simulink model "pcssp_PowerSupplies"  (R2020b)
settings: Solver=VariableStepAuto  StartTime=0.0  StopTime=10.0  RelTol=1e-3
model workspace (MAT data in the model file):
  PS_tp = Simulink.Parameter
  PS_tp.Value.currentLim = [0 55000 200000]
  PS_tp.Value.voltageLim = [1200 1050 1050]
  PS_tp.Value.VS3Vup = 2300
  PS_tp.Value.VS3Vlow = -2300
  PS_tp.DataType = 'struct'
  PS_tp.Dimensions = [1 1]
undefined symbols (not defined in the file or in its folder): PS_fp
settings Model: DataDictionary=pcssp_PowerSupplies.sldd  ParameterArgumentNames=PS_tp  OrderedModelArguments=off  Creator=ravenst1  LastModifiedBy=ravenst1
settings DebuggingCC: MergeDetectMultiDrivingBlocksExec=none
settings ModelReferenceCC: PropagateSignalLabelsOutOfModel=off

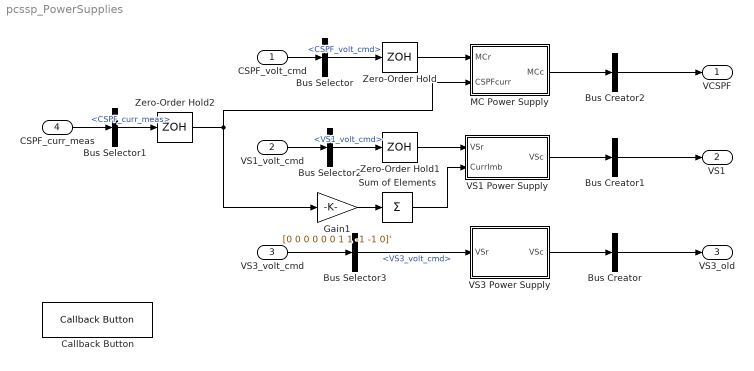
== system pcssp_PowerSupplies ==
  CSPF_volt_cmd : Inport  OutDataTypeStr=Bus: pcssp_PS_CSPF_volt_cmd  SampleTime=PS_fp.timing.dt
  VS1_volt_cmd : Inport  Port=2  OutDataTypeStr=Bus: pcssp_PS_VS1_volt_cmd  SampleTime=PS_fp.timing.dt
  VS3_volt_cmd : Inport  Port=3  OutDataTypeStr=Bus: pcssp_PS_VS3_volt_cmd  SampleTime=PS_fp.timing.dt
  CSPF_curr_meas : Inport  Port=4  OutDataTypeStr=Bus: pcssp_PS_CSPF_curr_meas  SampleTime=PS_fp.timing.dt
  Bus Creator : BusCreator  Inputs=1  OutDataTypeStr=Bus: pcssp_PS_VS3
      settings: InheritFromInputs=off
  Bus Creator1 : BusCreator  Inputs=1  OutDataTypeStr=Bus: pcssp_PS_VS1
      settings: InheritFromInputs=off
  Bus Creator2 : BusCreator  Inputs=1  OutDataTypeStr=Bus: pcssp_PS_VCSPF
      settings: InheritFromInputs=off
  Bus Selector : BusSelector  OutputSignals=CSPF_volt_cmd
  Bus Selector1 : BusSelector  OutputSignals=CSPF_curr_meas
  Bus Selector2 : BusSelector  OutputSignals=VS1_volt_cmd
  Bus Selector3 : BusSelector  OutputSignals=VS3_volt_cmd
  Callback Button : CallbackButton  ButtonText=Click for Module Documentation
      settings: ClickFcn=web(['file:///' which('PowerSupplies.html')])
  Gain1 : Gain  Gain=[0 0 0 0 0 0 1 1 -1 -1 0]'
  MC Power Supply : Subsystem
  Sum of Elements : Sum  Inputs=+
  VS1 Power Supply : Subsystem
  VS3 Power Supply : Subsystem
  Zero-Order Hold : ZeroOrderHold  SampleTime=PS_fp.timing.dt
  Zero-Order Hold1 : ZeroOrderHold  SampleTime=PS_fp.timing.dt
  Zero-Order Hold2 : ZeroOrderHold  SampleTime=PS_fp.timing.dt
  VCSPF : Outport  OutDataTypeStr=Bus: pcssp_PS_VCSPF
  VS1 : Outport  Port=2  OutDataTypeStr=Bus: pcssp_PS_VS1
  VS3_old : Outport  Port=3  OutDataTypeStr=Bus: pcssp_PS_VS3
  wires:
  VS3_volt_cmd/1 -> Bus Selector3/1
  Zero-Order Hold1/1 -> VS1 Power Supply/1(VSr)
  Sum of Elements/1 -> VS1 Power Supply/2(CurrImb)
  CSPF_curr_meas/1 -> Bus Selector1/1
  Zero-Order Hold2/1 -> Gain1/1, MC Power Supply/2(CSPFcurr)
  Zero-Order Hold/1 -> MC Power Supply/1(MCr)
  Gain1/1 -> Sum of Elements/1
  Bus Creator/1 -> VS3_old/1
  VS3 Power Supply/1(VSc) -> Bus Creator/1
  VS1 Power Supply/1(VSc) -> Bus Creator1/1
  Bus Creator1/1 -> VS1/1
  MC Power Supply/1(MCc) -> Bus Creator2/1
  Bus Creator2/1 -> VCSPF/1
  CSPF_volt_cmd/1 -> Bus Selector/1
  Bus Selector/1 -> Zero-Order Hold/1  "<CSPF_volt_cmd>"
  Bus Selector1/1 -> Zero-Order Hold2/1  "<CSPF_curr_meas>"
  VS1_volt_cmd/1 -> Bus Selector2/1
  Bus Selector2/1 -> Zero-Order Hold1/1  "<VS1_volt_cmd>"
  Bus Selector3/1 -> VS3 Power Supply/1(VSr)  "<VS3_volt_cmd>"

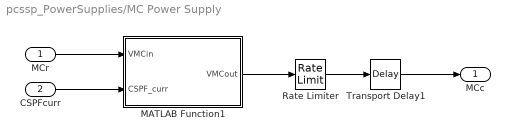
== system pcssp_PowerSupplies/MC Power Supply ==
  MCr : Inport
  CSPFcurr : Inport  Port=2
  MATLAB Function1 : MATLAB Function  TreatAsAtomicUnit=on  mask{currentLim=PS_tp.currentLim, voltageLim=PS_tp.voltageLim, nMConverters=PS_fp.nMConverters}
      mask prompts: currentLim "Current limits"; voltageLim "Voltage limits"; nMConverters "Number of CS/PF converters"
  Rate Limiter : RateLimiter  RisingSlewLimit=PS_fp.VMCpositiveSR  FallingSlewLimit=PS_fp.VMCnegativeSR  SampleTimeMode=inherited
  Transport Delay1 : TransportDelay  DelayTime=PS_fp.VMCtaud
  MCc : Outport
  wires:
  MCr/1 -> MATLAB Function1/1(VMCin)
  CSPFcurr/1 -> MATLAB Function1/2(CSPF_curr)
  MATLAB Function1/1(VMCout) -> Rate Limiter/1
  Rate Limiter/1 -> Transport Delay1/1
  Transport Delay1/1 -> MCc/1

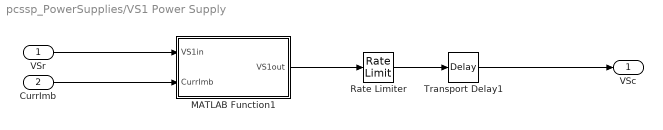
== system pcssp_PowerSupplies/VS1 Power Supply ==
  VSr : Inport
  CurrImb : Inport  Port=2
  MATLAB Function1 : MATLAB Function  TreatAsAtomicUnit=on  mask{currentLim=PS_tp.currentLim, voltageLim=PS_tp.voltageLim, nVS1Converters=PS_fp.nVS1Converters}
      mask prompts: currentLim "Current limit"; voltageLim "Voltage limit"; nVS1Converters "Number of VS1 converters"
  Rate Limiter : RateLimiter  RisingSlewLimit=PS_fp.VS1positiveSR  FallingSlewLimit=PS_fp.VS1negativeSR  SampleTimeMode=inherited
  Transport Delay1 : TransportDelay  DelayTime=PS_fp.VS1taud
  VSc : Outport
  wires:
  CurrImb/1 -> MATLAB Function1/2(CurrImb)
  VSr/1 -> MATLAB Function1/1(VS1in)
  Transport Delay1/1 -> VSc/1
  MATLAB Function1/1(VS1out) -> Rate Limiter/1
  Rate Limiter/1 -> Transport Delay1/1

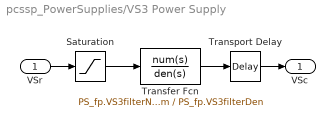
== system pcssp_PowerSupplies/VS3 Power Supply ==
  VSr : Inport
  Saturation : Saturate  UpperLimit=PS_tp.VS3Vup  LowerLimit=PS_tp.VS3Vlow
  Transfer Fcn : TransferFcn  Numerator=PS_fp.VS3filterNum  Denominator=PS_fp.VS3filterDen
  Transport Delay : TransportDelay  DelayTime=PS_fp.VS3taud
  VSc : Outport
  wires:
  VSr/1 -> Saturation/1
  Transport Delay/1 -> VSc/1
  Transfer Fcn/1 -> Transport Delay/1
  Saturation/1 -> Transfer Fcn/1

== matlab function pcssp_PowerSupplies/VS1 Power Supply/MATLAB Function1 ==
  data: VS1in input; VS1out output; CurrImb input; currentLim parameter; voltageLim parameter; nVS1Converters parameter
function VS1out  = fcn(VS1in, CurrImb, currentLim, voltageLim, nVS1Converters)
VoltageLimits = interp1(currentLim,[voltageLim.*nVS1Converters]',abs(CurrImb));
VS1in = min(VS1in,VoltageLimits);
VS1out = max(VS1in,-VoltageLimits);

== matlab function pcssp_PowerSupplies/MC Power Supply/MATLAB Function1 ==
  data: VMCin input; VMCout output; CSPF_curr input; currentLim parameter; voltageLim parameter; nMConverters parameter
function VMCout  = fcn(VMCin, CSPF_curr, currentLim, voltageLim, nMConverters)
VoltageLimits = zeros(11,1);
for ii=1:11
    VoltageLimits(ii) = interp1(currentLim,[voltageLim.*nMConverters(ii)]',abs(CSPF_curr(ii)));
end
VMCin = min(VMCin,VoltageLimits);
VMCout = max(VMCin,-VoltageLimits);
